simulink model "vanderpol"  (Simulink 7.9)
settings: Solver=ode45  StartTime=0.0  StopTime=10.0  RelTol=1e-3
values from neighbouring files (symbols this model uses):
  epsilon = 1    [skrypt.m]
undefined symbols (not defined in the file or in its folder): x_1, x_2
settings Model: Creator=student  LastModifiedBy=student

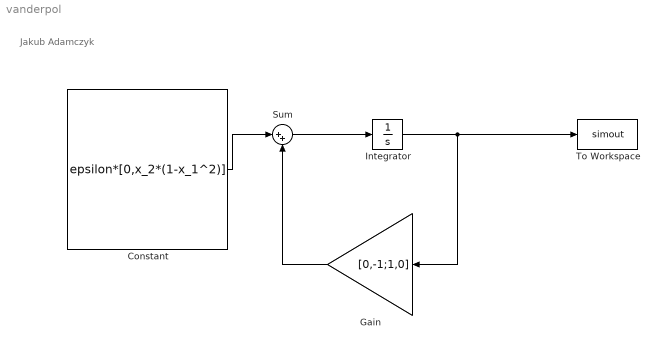
== system vanderpol ==
  note: Jakub Adamczyk
  Constant : Constant  Value=epsilon*[0,x_2*(1-x_1^2)]
  Gain : Gain  Gain=[0,-1;1,0]
  Integrator : Integrator
  Sum : Sum  Inputs=|++
  To Workspace : ToWorkspace  VariableName=simout  SampleTime=-1  SaveFormat=Timeseries
  wires:
  Integrator/1 -> Gain/1, To Workspace/1
  Sum/1 -> Integrator/1
  Gain/1 -> Sum/2
  Constant/1 -> Sum/1
